simulink model "am_sys4"  (Simulink 3.00)
settings: Solver=ode45  StartTime=0.0  StopTime=999999  MaxStep=0.001  RelTol=1e-3  AbsTol=1e-3
settings Model: SaveTime=off  SaveOutput=off

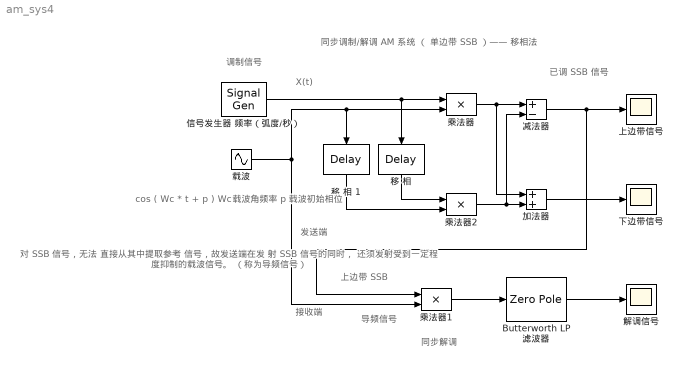
== system am_sys4 ==
  note: 同步解调
  note: 导频信号
  note: 上边带 SSB
  note: 发送端
  note: 接收端
  note: cos ( Wc * t + p )
      | Wc 载波角频率
      | p 载波初始相位
  note: 已调 SSB 信号
  note: X(t)
  note: 调制信号
  note: 对 SSB 信号，无法
      | 直接从其中提取参考
      | 信号，故发送端在发
      | 射 SSB 信号的同时，
      | 还须发射受到一定程
      | 度抑制的载波信号。
      | （称为导频信号）
  note: 同步调制/解调 AM 系统 （ 单边带 SSB ）—— 移相法
  Butterworth LP 滤波器 : ZeroPole  Zeros=z  Poles=p  Gain=k  mask(buttap){@1=15, @2=4}
      mask prompts: @1 "Cutoff frequency (rad/sec)"; @2 "Order"
      mask help:
      | Analog Butterworth low pass filter.
      |
      | (Requires Signal Processing Toolbox)
      mask init:
      | [z,p,k]=buttap(@2); z=@1*z; p=@1*p; k=real(prod(-p)); [num,den]=zp2tf(z,p,k); w=logspace(log10(@1/10),log10(10*@1),20); h=freqs(num,den,w);
      mask Help: Butterworth low pass filter using MATLAB's butter command.
      mask Display: plot(20*log10(w),20*log10(abs(h)))
  乘法器 : Product  Inputs=2  SaturateOnIntegerOverflow=on
      mask Type: 乘法器
      mask Description: 乘法器
      mask Display: plot([0 1],[1 0],[0 1],[0 1]);
  乘法器1 : Product  Inputs=2  SaturateOnIntegerOverflow=on
      mask Type: 乘法器
      mask Description: 乘法器
      mask Display: plot([0 1],[1 0],[0 1],[0 1]);
  乘法器2 : Product  Inputs=2  SaturateOnIntegerOverflow=on
      mask Type: 乘法器
      mask Description: 乘法器
      mask Display: plot([0 1],[1 0],[0 1],[0 1]);
  加法器 : Sum  Inputs=++  SaturateOnIntegerOverflow=on
  减法器 : Sum  Inputs=+-  SaturateOnIntegerOverflow=on
  解调信号 : Scope
      settings: TimeRange=1.000000  YMin=-1  YMax=1  SaveToWorkspace=off  SaveName=ScopeData  DataFormat=Matrix
  上边带信号 : Scope
      settings: TimeRange=1.000000  YMin=-2  YMax=2  SaveToWorkspace=off  SaveName=ScopeData  DataFormat=Matrix
  下边带信号 : Scope
      settings: TimeRange=1.000000  YMin=-2  YMax=2  SaveToWorkspace=off  SaveName=ScopeData  DataFormat=Matrix
  信号发生器 频率（弧度/秒） : SignalGenerator  WaveForm=sine  Amplitude=1.000000  Frequency=10.000000  Units=rad/sec
  移 相 : TransportDelay  Orientation=down  DelayTime=0.25/(W/(2*pi))  InitialInput=0  BufferSize=1024  mask(90度移相){@1=10}
      mask prompts: @1 "输入信号的角频率（Rad/s）："
      mask help: 90度移相
      mask init:
      | W=@1;
      mask Display: disp('90度')
  移 相 1 : TransportDelay  Orientation=down  DelayTime=0.25/(W/(2*pi))  InitialInput=0  BufferSize=1024  mask(90度移相){@1=100}
      mask prompts: @1 "输入信号的角频率（Rad/s）："
      mask help: 90度移相
      mask init:
      | W=@1;
      mask Display: disp('90度')
  载波 : Sin  Amplitude=1  Frequency=100  Phase=0  SampleTime=0.001
  wires:
  乘法器1/1 -> Butterworth LP 滤波器/1
  Butterworth LP 滤波器/1 -> 解调信号/1
  信号发生器 频率（弧度/秒）/1 -> 移 相/1, 乘法器/1
  移 相 1/1 -> 乘法器2/2
  移 相/1 -> 乘法器2/1
  加法器/1 -> 下边带信号/1
  乘法器/1 -> 减法器/1, 加法器/1
  乘法器2/1 -> 加法器/2, 减法器/2
  减法器/1 -> 上边带信号/1, 乘法器1/1
  载波/1 -> 乘法器/2, 移 相 1/1, 乘法器1/2
